simulink model "Simulacion2"  (R2023a)
settings: Solver=VariableStepAuto  StartTime=0.0  StopTime=12  RelTol=1e-3
libraries: spsDCVoltageSourceLib x2, spsDCMachineLib x1, sps_lib x1
settings Model: Creator=alexa  LastModifiedBy=alexa

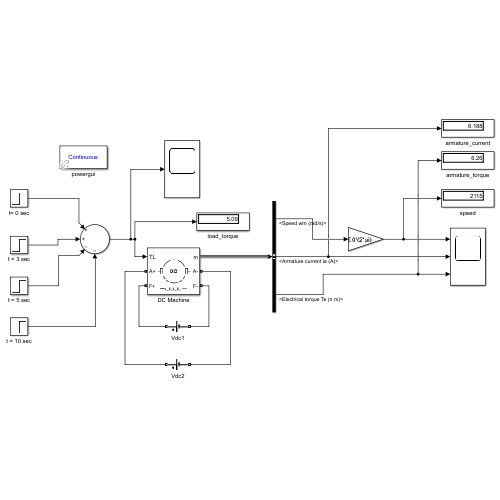
[thumbnail: Simulink's stored preview of the top-level diagram]
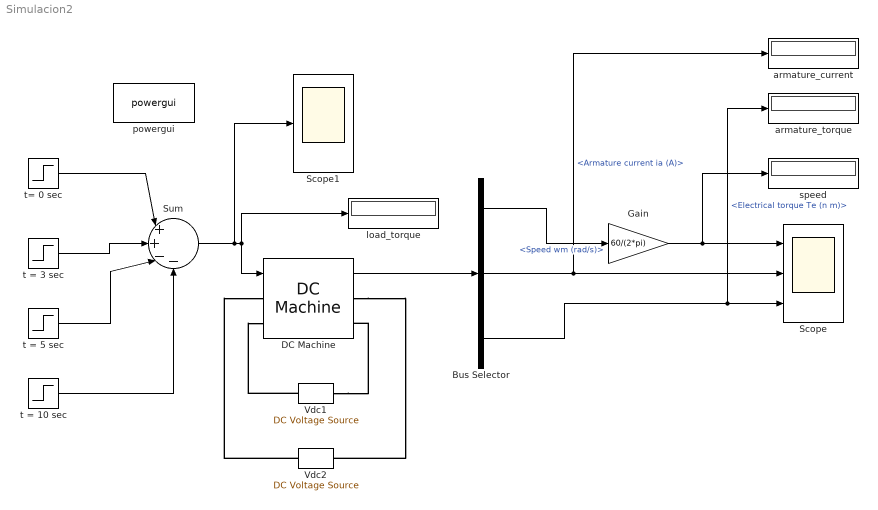
== system Simulacion2 ==
  Bus Selector : BusSelector  OutputSignals=Speed wm (rad/s),Armature current ia (A),Electrical torque Te (n m)
  "DC Machine " : spsDCMachineLib/DC Machine  PresetModel=No  MechanicalLoad=Torque TL  FieldType=Wound  ShowDetailedParameters=on  MeasurementBus=off  RLa=[2.581 0.028]  RLf=[281.2 156]  Laf=0.9483  MachineConstant=Torque constant (N.m/A)  Ke=1.8  Kt=1.8  J=0.02215  Bm=0.002953  Tf=0.5161  w0=1  Ifinit=1.06685633001422  TsPowergui=0  TsBlock=-1
  Gain : Gain  Gain=60/(2*pi)
  Scope : Scope  NumInputPorts=3
  Scope1 : Scope
  Sum : Sum  Inputs=|++--
  "Vdc1 " : spsDCVoltageSourceLib/DC Voltage Source  Amplitude=300  Measurements=None
  Vdc2 : spsDCVoltageSourceLib/DC Voltage Source  Amplitude=240  Measurements=None
  armature_current : Display
  armature_torque : Display
  load_torque : Display
  powergui : sps_lib/powergui  Priority=1  SimulationMode=Continuous  SampleTime=50e-6  frequency=60  Iterations=50  frequencyindice=0  Pbase=100e6  ErrMax=1e-4  UnitsV=kV  UnitsW=MW  buscounter=0  FunctionMessages=off  echomessages=off  EnableUseOfTLC=off  CurrentSourceSwitches=off  DisableSnubberDevices=off  DisableRonSwitches=off  DisableVfSwitches=off  DisplayEquations=off  AutomaticDiscreteSolvers=off  SolverType=Tustin/Backward Euler (TBE)  Interpol=off  ExternalGateDelay=off  methode=off  Ts=100  x0status=blocks  SPID=on  SwTol=0  HookPort=off  NonlinearTolerance=1e-4  nMaxIteration=100  ContinueOnMaxIteration=off  RestoreLinks=warning  ResistiveCurrentMeasurement=off  Frange=[0:2:500]  Ylog=off  Xlog=on  ShowGrid=off  save=off  variable=ZData  structure=0  ZoomFFT=off  StartTime=0.0  cycles=1  DisplayStyle=1  fundamental=60  FreqAxis=off  MaxFrequency=1000  frequencyindicesteady=1  RmsSteady=1  display=off
  speed : Display
  t = 10 sec : Step  Time=10  After=5.09  SampleTime=0
  t = 3 sec : Step  Time=3  After=20.36  SampleTime=0
  t = 5 sec : Step  Time=5  After=10.18  SampleTime=0
  t= 0 sec : Step  Time=0  After=0  SampleTime=0
  wires:
  "DC Machine "/1 -> Bus Selector/1
  Bus Selector/1 -> Gain/1  "<Speed wm (rad/s)>"
  Bus Selector/2 -> armature_current/1, Scope/2  "<Armature current ia (A)>"
  Bus Selector/3 -> Scope/3, armature_torque/1  "<Electrical torque Te (n m)>"
  Gain/1 -> speed/1, Scope/1
  t= 0 sec/1 -> Sum/1
  t = 3 sec/1 -> Sum/2
  t = 5 sec/1 -> Sum/3
  t = 10 sec/1 -> Sum/4
  Sum/1 -> Scope1/1, "DC Machine "/1, load_torque/1
  connections:
  "Vdc1 "/RConn1 -- "DC Machine "/LConn2
  "Vdc1 "/LConn1 -- "DC Machine "/RConn2
  "DC Machine "/RConn1 -- Vdc2/LConn1
  Vdc2/RConn1 -- "DC Machine "/LConn1
